simulink model "CTC"  (R2022b)
settings: Solver=VariableStepAuto  StartTime=0.0  StopTime=30  RelTol=1e-3
model workspace (MATLAB code in the model file):
  | % Simscape(TM) Multibody(TM) version: 7.3
  | 
  | % This is a model data file derived from a Simscape Multibody Import XML file using the smimport function.
  | % The data in this file sets the block parameter values in an imported Simscape Multibody model.
  | % For more information on this file, see the smimport function help page in the Simscape Multibody documentation.
  | % You can modify numerical values, but avoid any other changes to this file.
  | % Do not add code to this file. Do not edit the physical units shown in comments.
  | 
  | %%%VariableName:smiData
  | 
  | 
  | %============= RigidTransform =============%
  | 
  | %Initialize the RigidTransform structure array by filling in null values.
  | smiData.RigidTransform(98).translation = [0.0 0.0 0.0];
  | smiData.RigidTransform(98).angle = 0.0;
  | smiData.RigidTransform(98).axis = [0.0 0.0 0.0];
  | smiData.RigidTransform(98).ID = '';
  | 
  | %Translation Method - Cartesian
  | %Rotation Method - Arbitrary Axis
  | smiData.RigidTransform(1).translation = [0 19.999999999999989 175];  % mm
  | smiData.RigidTransform(1).angle = 2.0943951023931953;  % rad
  | smiData.RigidTransform(1).axis = [0.57735026918962584 -0.57735026918962584 0.57735026918962584];
  | smiData.RigidTransform(1).ID = 'B[UpperLeg_2:Upper_Leg-1:-:UpperLeg_2:Joint_1-1]';
  | 
  | %Translation Method - Cartesian
  | %Rotation Method - Arbitrary Axis
  | smiData.RigidTransform(2).translation = [-10.000000000089699 -1.8161827597396041e-10 -1.8518164779379731e-10];  % mm
  | smiData.RigidTransform(2).angle = 2.0943951023931953;  % rad
  | smiData.RigidTransform(2).axis = [0.57735026918962618 0.57735026918962562 0.5773502691896254];
  | smiData.RigidTransform(2).ID = 'F[UpperLeg_2:Upper_Leg-1:-:UpperLeg_2:Joint_1-1]';
  | 
  | %Translation Method - Cartesian
  | %Rotation Method - Arbitrary Axis
  | smiData.RigidTransform(3).translation = [117.00317547305409 9.9999999999999947 -56.489637028919212];  % mm
  | smiData.RigidTransform(3).angle = 0.52359877559830381;  % rad
  | smiData.RigidTransform(3).axis = [-0 -1 0];
  | smiData.RigidTransform(3).ID = 'B[Base_3:�?-1:-:Base_3:Joint_1-1]';
  | 
  | %Translation Method - Cartesian
  | %Rotation Method - Arbitrary Axis
  | smiData.RigidTransform(4).translation = [107.42304845737816 8.9706091443986224e-09 1.015528994230408e-08];  % mm
  | smiData.RigidTransform(4).angle = 2.0943951023930776;  % rad
  | smiData.RigidTransform(4).axis = [-0.57735026918962873 -0.57735026918958643 0.57735026918966204];
  | smiData.RigidTransform(4).ID = 'F[Base_3:�?-1:-:Base_3:Joint_1-1]';
  | 
  | %Translation Method - Cartesian
  | %Rotation Method - Arbitrary Axis
  | smiData.RigidTransform(5).translation = [-21.650635094607303 9.9999999999995097 108.66580753731172];  % mm
  | smiData.RigidTransform(5).angle = 3.1415926535897865;  % rad
  | smiData.RigidTransform(5).axis = [-0.96592582628906776 -8.8781377035549872e-16 0.25881904510252285];
  | smiData.RigidTransform(5).ID = 'B[Base_3:�?-1:-:Base_3:Joint_1-4]';
  | 
  | %Translation Method - Cartesian
  | %Rotation Method - Arbitrary Axis
  | smiData.RigidTransform(6).translation = [83.282032288587871 4.5821799687928433e-09 1.1489191820146516e-09];  % mm
  | smiData.RigidTransform(6).angle = 2.094395102393289;  % rad
  | smiData.RigidTransform(6).axis = [-0.57735026918951493 -0.57735026918965693 0.57735026918970545];
  | smiData.RigidTransform(6).ID = 'F[Base_3:�?-1:-:Base_3:Joint_1-4]';
  | 
  | %Translation Method - Cartesian
  | %Rotation Method - Arbitrary Axis
  | smiData.RigidTransform(7).translation = [-76.282032302753606 10.000000000000147 -73.082903768653054];  % mm
  | smiData.RigidTransform(7).angle = 2.094395102393197;  % rad
  | smiData.RigidTransform(7).axis = [0.57735026918962462 0.57735026918962629 0.5773502691896264];
  | smiData.RigidTransform(7).ID = 'B[Base_3:�?-1:-:Base_3:Joint_1-5]';
  | 
  | %Translation Method - Cartesian
  | %Rotation Method - Arbitrary Axis
  | smiData.RigidTransform(8).translation = [-76.28203231342502 8.5679736105508616e-09 -5.5658047997319685e-09];  % mm
  | smiData.RigidTransform(8).angle = 2.0943951023931096;  % rad
  | smiData.RigidTransform(8).axis = [0.57735026918957733 0.5773502691895972 0.57735026918970267];
  | smiData.RigidTransform(8).ID = 'F[Base_3:�?-1:-:Base_3:Joint_1-5]';
  | 
  | %Translation Method - Cartesian
  | %Rotation Method - Arbitrary Axis
  | smiData.RigidTransform(9).translation = [-18.655092795423545 178.99125127896585 252.03989417796402];  % mm
  | smiData.RigidTransform(9).angle = 2.094395102393197;  % rad
  | smiData.RigidTransform(9).axis = [0.5773502691896264 -0.57735026918962462 0.5773502691896264];
  | smiData.RigidTransform(9).ID = 'B[LowerLeg_Assembly#2-2:-:x?-10]';
  | 
  | %Translation Method - Cartesian
  | %Rotation Method - Arbitrary Axis
  | smiData.RigidTransform(10).translation = [3.0000000000001261 -4.0059067174524898e-12 -5.8264504332328215e-13];  % mm
  | smiData.RigidTransform(10).angle = 2.0943951023931953;  % rad
  | smiData.RigidTransform(10).axis = [0.57735026918962584 0.57735026918962584 0.57735026918962584];
  | smiData.RigidTransform(10).ID = 'F[LowerLeg_Assembly#2-2:-:x?-10]';
  | 
  | %Translation Method - Cartesian
  | %Rotation Method - Arbitrary Axis
  | smiData.RigidTransform(11).translation = [0 5.0000000000000044 0];  % mm
  | smiData.RigidTransform(11).angle = 2.0943951023931957;  % rad
  | smiData.RigidTransform(11).axis = [-0.57735026918962584 -0.57735026918962573 -0.57735026918962573];
  | smiData.RigidTransform(11).ID = 'B[UpperLeg_2-3:Joint_1-1:-:x?-10]';
  | 
  | %Translation Method - Cartesian
  | %Rotation Method - Arbitrary Axis
  | smiData.RigidTransform(12).translation = [-1.2569500995596172e-11 5.2091847198853705 -31.573159401015047];  % mm
  | smiData.RigidTransform(12).angle = 2.0943951023870682;  % rad
  | smiData.RigidTransform(12).axis = [-0.5773502691928436 -0.57735026918758314 0.57735026918845045];
  | smiData.RigidTransform(12).ID = 'F[UpperLeg_2-3:Joint_1-1:-:x?-10]';
  | 
  | %Translation Method - Cartesian
  | %Rotation Method - Arbitrary Axis
  | smiData.RigidTransform(13).translation = [31.999999999999918 5.0000000000000044 0];  % mm
  | smiData.RigidTransform(13).angle = 2.0943951023931953;  % rad
  | smiData.RigidTransform(13).axis = [0.57735026918962584 -0.57735026918962584 0.57735026918962584];
  | smiData.RigidTransform(13).ID = 'B[UpperLeg_2-5:Joint_1-1:-:x?-11]';
  | 
  | %Translation Method - Cartesian
  | %Rotation Method - Arbitrary Axis
  | smiData.RigidTransform(14).translation = [-7.9273054803145348e-11 1.3585044680166562e-11 -8.760761212378511e-11];  % mm
  | smiData.RigidTransform(14).angle = 2.0943951023967697;  % rad
  | smiData.RigidTransform(14).axis = [0.5773502691867648 0.57735026919081722 0.57735026919129528];
  | smiData.RigidTransform(14).ID = 'F[UpperLeg_2-5:Joint_1-1:-:x?-11]';
  | 
  | %Translation Method - Cartesian
  | %Rotation Method - Arbitrary Axis
  | smiData.RigidTransform(15).translation = [-32.000000000000028 5.0000000000000044 0];  % mm
  | smiData.RigidTransform(15).angle = 2.0943951023931953;  % rad
  | smiData.RigidTransform(15).axis = [0.57735026918962584 -0.57735026918962584 0.57735026918962584];
  | smiData.RigidTransform(15).ID = 'B[UpperLeg_2-5:Joint_1-1:-:x?-12]';
  | 
  | %Translation Method - Cartesian
  | %Rotation Method - Arbitrary Axis
  | smiData.RigidTransform(16).translation = [-7.9191762745372911e-11 1.3376425944582028e-11 -8.7773195960719397e-11];  % mm
  | smiData.RigidTransform(16).angle = 2.0943951023967693;  % rad
  | smiData.RigidTransform(16).axis = [0.57735026918676491 0.57735026919081711 0.57735026919129517];
  | smiData.RigidTransform(16).ID = 'F[UpperLeg_2-5:Joint_1-1:-:x?-12]';
  | 
  | %Translation Method - Cartesian
  | %Rotation Method - Arbitrary Axis
  | smiData.RigidTransform(17).translation = [130.75000000000338 55.000000000000355 -100.89195954089351];  % mm
  | smiData.RigidTransform(17).angle = 3.1415926535897878;  % rad
  | smiData.RigidTransform(17).axis = [0.96592582628906765 -7.5033484398435492e-16 -0.25881904510252302];
  | smiData.RigidTransform(17).ID = 'B[Base-1:-:UpperLeg_2-5:Upper_Leg-1]';
  | 
  | %Translation Method - Cartesian
  | %Rotation Method - Arbitrary Axis
  | smiData.RigidTransform(18).translation = [6.2172489379008766e-15 -12.000000000004182 -6.5725203057809267e-14];  % mm
  | smiData.RigidTransform(18).angle = 2.094395102393197;  % rad
  | smiData.RigidTransform(18).axis = [0.57735026918962629 -0.5773502691896254 0.57735026918962562];
  | smiData.RigidTransform(18).ID = 'F[Base-1:-:UpperLeg_2-5:Upper_Leg-1]';
  | 
  | %Translation Method - Cartesian
  | %Rotation Method - Arbitrary Axis
  | smiData.RigidTransform(19).translation = [353.38874943283707 174.99125127896704 252.03989417796384];  % mm
  | smiData.RigidTransform(19).angle = 2.0943951023931939;  % rad
  | smiData.RigidTransform(19).axis = [-0.57735026918962529 -0.57735026918962695 -0.57735026918962518];
  | smiData.RigidTransform(19).ID = 'B[LowerLeg_Assembly#2-1:-:Base_3-1:Joint_1-5]';
  | 
  | %Translation Method - Cartesian
  | %Rotation Method - Arbitrary Axis
  | smiData.RigidTransform(20).translation = [-32.00000001037607 2.0000000085989118 -5.446665340969048e-09];  % mm
  | smiData.RigidTransform(20).angle = 2.09439510239261;  % rad
  | smiData.RigidTransform(20).axis = [0.57735026918943078 -0.57735026918942933 0.5773502691900172];
  | smiData.RigidTransform(20).ID = 'F[LowerLeg_Assembly#2-1:-:Base_3-1:Joint_1-5]';
  | 
  | %Translation Method - Cartesian
  | %Rotation Method - Arbitrary Axis
  | smiData.RigidTransform(21).translation = [-32.000000000000028 5.000000000000032 0];  % mm
  | smiData.RigidTransform(21).angle = 2.0943951023931953;  % rad
  | smiData.RigidTransform(21).axis = [0.57735026918962584 -0.57735026918962584 0.57735026918962584];
  | smiData.RigidTransform(21).ID = 'B[UpperLeg_2-3:Joint_1-1:-:LowerLeg_Assembly#2-1]';
  | 
  | %Translation Method - Cartesian
  | %Rotation Method - Arbitrary Axis
  | smiData.RigidTransform(22).translation = [-18.655092795320627 181.99125127897832 252.03989417784715];  % mm
  | smiData.RigidTransform(22).angle = 2.0943951023881247;  % rad
  | smiData.RigidTransform(22).axis = [0.57735026918793542 -0.57735026919325916 0.57735026918768262];
  | smiData.RigidTransform(22).ID = 'F[UpperLeg_2-3:Joint_1-1:-:LowerLeg_Assembly#2-1]';
  | 
  | %Translation Method - Cartesian
  | %Rotation Method - Arbitrary Axis
  | smiData.RigidTransform(23).translation = [353.38874943283662 174.99125127896701 252.03989417796402];  % mm
  | smiData.RigidTransform(23).angle = 2.0943951023931939;  % rad
  | smiData.RigidTransform(23).axis = [-0.57735026918962529 -0.57735026918962706 -0.57735026918962495];
  | smiData.RigidTransform(23).ID = 'B[LowerLeg_Assembly#2-2:-:Base_3-1:Joint_1-5]';
  | 
  | %Translation Method - Cartesian
  | %Rotation Method - Arbitrary Axis
  | smiData.RigidTransform(24).translation = [31.999999989623838 2.000000008599276 -5.4573305874328071e-09];  % mm
  | smiData.RigidTransform(24).angle = 2.0943951023926095;  % rad
  | smiData.RigidTransform(24).axis = [0.57735026918943044 -0.57735026918942922 0.57735026919001764];
  | smiData.RigidTransform(24).ID = 'F[LowerLeg_Assembly#2-2:-:Base_3-1:Joint_1-5]';
  | 
  | %Translation Method - Cartesian
  | %Rotation Method - Arbitrary Axis
  | smiData.RigidTransform(25).translation = [31.999999999999972 5.000000000000032 0];  % mm
  | smiData.RigidTransform(25).angle = 2.0943951023931953;  % rad
  | smiData.RigidTransform(25).axis = [0.57735026918962584 -0.57735026918962584 0.57735026918962584];
  | smiData.RigidTransform(25).ID = 'B[UpperLeg_2-3:Joint_1-1:-:LowerLeg_Assembly#2-2]';
  | 
  | %Translation Method - Cartesian
  | %Rotation Method - Arbitrary Axis
  | smiData.RigidTransform(26).translation = [-18.655092795316818 181.99125127897861 252.03989417784709];  % mm
  | smiData.RigidTransform(26).angle = 2.0943951023881242;  % rad
  | smiData.RigidTransform(26).axis = [0.57735026918793531 -0.57735026919325916 0.57735026918768284];
  | smiData.RigidTransform(26).ID = 'F[UpperLeg_2-3:Joint_1-1:-:LowerLeg_Assembly#2-2]';
  | 
  | %Translation Method - Cartesian
  | %Rotation Method - Arbitrary Axis
  | smiData.RigidTransform(27).translation = [-18.655092795423545 174.99125127896542 252.03989417796402];  % mm
  | smiData.RigidTransform(27).angle = 2.0943951023931935;  % rad
  | smiData.RigidTransform(27).axis = [-0.57735026918962518 -0.57735026918962695 -0.57735026918962518];
  | smiData.RigidTransform(27).ID = 'B[LowerLeg_Assembly#2-3:-:Base_3-1:Joint_1-4]';
  | 
  | %Translation Method - Cartesian
  | %Rotation Method - Arbitrary Axis
  | smiData.RigidTransform(28).translation = [31.999999986078205 -1.9999999955871002 8.734324374870539e-10];  % mm
  | smiData.RigidTransform(28).angle = 2.094395102390521;  % rad
  | smiData.RigidTransform(28).axis = [-0.57735026918873433 -0.57735026918873378 -0.5773502691914093];
  | smiData.RigidTransform(28).ID = 'F[LowerLeg_Assembly#2-3:-:Base_3-1:Joint_1-4]';
  | 
  | %Translation Method - Cartesian
  | %Rotation Method - Arbitrary Axis
  | smiData.RigidTransform(29).translation = [-31.999999999999972 4.9999999999998934 0];  % mm
  | smiData.RigidTransform(29).angle = 2.0943951023931953;  % rad
  | smiData.RigidTransform(29).axis = [0.57735026918962584 -0.57735026918962584 0.57735026918962584];
  | smiData.RigidTransform(29).ID = 'B[UpperLeg_2-4:Joint_1-1:-:LowerLeg_Assembly#2-3]';
  | 
  | %Translation Method - Cartesian
  | %Rotation Method - Arbitrary Axis
  | smiData.RigidTransform(30).translation = [353.38874943270537 181.99125127899549 252.03989417800804];  % mm
  | smiData.RigidTransform(30).angle = 2.0943951023971508;  % rad
  | smiData.RigidTransform(30).axis = [0.57735026919094412 -0.57735026918594667 0.5773502691919864];
  | smiData.RigidTransform(30).ID = 'F[UpperLeg_2-4:Joint_1-1:-:LowerLeg_Assembly#2-3]';
  | 
  | %Translation Method - Cartesian
  | %Rotation Method - Arbitrary Axis
  | smiData.RigidTransform(31).translation = [-18.655092795423602 174.99125127896565 252.03989417796413];  % mm
  | smiData.RigidTransform(31).angle = 2.0943951023931935;  % rad
  | smiData.RigidTransform(31).axis = [-0.57735026918962518 -0.57735026918962695 -0.57735026918962518];
  | smiData.RigidTransform(31).ID = 'B[LowerLeg_Assembly#2-4:-:Base_3-1:Joint_1-4]';
  | 
  | %Translation Method - Cartesian
  | %Rotation Method - Arbitrary Axis
  | smiData.RigidTransform(32).translation = [-32.000000013922282 -1.9999999955870065 8.6944784705167422e-10];  % mm
  | smiData.RigidTransform(32).angle = 2.094395102390521;  % rad
  | smiData.RigidTransform(32).axis = [-0.57735026918873411 -0.57735026918873411 -0.57735026919140886];
  | smiData.RigidTransform(32).ID = 'F[LowerLeg_Assembly#2-4:-:Base_3-1:Joint_1-4]';
  | 
  | %Translation Method - Cartesian
  | %Rotation Method - Arbitrary Axis
  | smiData.RigidTransform(33).translation = [32.000000000000028 -4.5000000000001705 0];  % mm
  | smiData.RigidTransform(33).angle = 2.0943951023931953;  % rad
  | smiData.RigidTransform(33).axis = [0.57735026918962584 -0.57735026918962584 0.57735026918962584];
  | smiData.RigidTransform(33).ID = 'B[UpperLeg_2-4:Joint_1-1:-:LowerLeg_Assembly#2-4]';
  | 
  | %Translation Method - Cartesian
  | %Rotation Method - Arbitrary Axis
  | smiData.RigidTransform(34).translation = [353.38874943278768 172.49125127899504 252.03989417802512];  % mm
  | smiData.RigidTransform(34).angle = 2.0943951023971494;  % rad
  | smiData.RigidTransform(34).axis = [0.57735026919094379 -0.57735026918594712 0.57735026919198651];
  | smiData.RigidTransform(34).ID = 'F[UpperLeg_2-4:Joint_1-1:-:LowerLeg_Assembly#2-4]';
  | 
  | %Translation Method - Cartesian
  | %Rotation Method - Arbitrary Axis
  | smiData.RigidTransform(35).translation = [-18.655092795423659 174.99125127896588 252.03989417796402];  % mm
  | smiData.RigidTransform(35).angle = 2.0943951023931935;  % rad
  | smiData.RigidTransform(35).axis = [-0.57735026918962518 -0.57735026918962695 -0.57735026918962518];
  | smiData.RigidTransform(35).ID = 'B[LowerLeg_Assembly#2-5:-:Base_3-1:Joint_1-1]';
  | 
  | %Translation Method - Cartesian
  | %Rotation Method - Arbitrary Axis
  | smiData.RigidTransform(36).translation = [-31.999999996925382 2.0000000089001038 9.9767270000938879e-09];  % mm
  | smiData.RigidTransform(36).angle = 2.0943951023932001;  % rad
  | smiData.RigidTransform(36).axis = [0.57735026918962729 -0.57735026918962384 0.57735026918962629];
  | smiData.RigidTransform(36).ID = 'F[LowerLeg_Assembly#2-5:-:Base_3-1:Joint_1-1]';
  | 
  | %Translation Method - Cartesian
  | %Rotation Method - Arbitrary Axis
  | smiData.RigidTransform(37).translation = [-18.655092795423542 174.99125127896585 252.03989417796407];  % mm
  | smiData.RigidTransform(37).angle = 2.0943951023931935;  % rad
  | smiData.RigidTransform(37).axis = [-0.57735026918962518 -0.57735026918962695 -0.57735026918962518];
  | smiData.RigidTransform(37).ID = 'B[LowerLeg_Assembly#2-6:-:Base_3-1:Joint_1-1]';
  | 
  | %Translation Method - Cartesian
  | %Rotation Method - Arbitrary Axis
  | smiData.RigidTransform(38).translation = [32.000000003094932 2.0000000089002699 1.0007141781898099e-08];  % mm
  | smiData.RigidTransform(38).angle = 2.0943951023932006;  % rad
  | smiData.RigidTransform(38).axis = [0.5773502691896274 -0.5773502691896244 0.57735026918962551];
  | smiData.RigidTransform(38).ID = 'F[LowerLeg_Assembly#2-6:-:Base_3-1:Joint_1-1]';
  | 
  | %Translation Method - Cartesian
  | %Rotation Method - Arbitrary Axis
  | smiData.RigidTransform(39).translation = [-7.9999999999974776 54.999999999999467 163.67880131526533];  % mm
  | smiData.RigidTransform(39).angle = 2.0943951023931975;  % rad
  | smiData.RigidTransform(39).axis = [-0.57735026918962351 -0.57735026918962651 0.57735026918962717];
  | smiData.RigidTransform(39).ID = 'B[Base-1:-:UpperLeg_2-4:Upper_Leg-1]';
  | 
  | %Translation Method - Cartesian
  | %Rotation Method - Arbitrary Axis
  | smiData.RigidTransform(40).translation = [-2.6645352591003757e-15 2 -1.6620038678638593e-13];  % mm
  | smiData.RigidTransform(40).angle = 2.0943951023931953;  % rad
  | smiData.RigidTransform(40).axis = [0.57735026918962584 -0.57735026918962595 0.57735026918962562];
  | smiData.RigidTransform(40).ID = 'F[Base-1:-:UpperLeg_2-4:Upper_Leg-1]';
  | 
  | %Translation Method - Cartesian
  | %Rotation Method - Arbitrary Axis
  | smiData.RigidTransform(41).translation = [-137.75000000000676 54.999999999998977 -88.767603887906532];  % mm
  | smiData.RigidTransform(41).angle = 3.1415926535897931;  % rad
  | smiData.RigidTransform(41).axis = [-0.96592582628906787 2.1099173714894905e-17 -0.25881904510252235];
  | smiData.RigidTransform(41).ID = 'B[Base-1:-:UpperLeg_2-3:Upper_Leg-1]';
  | 
  | %Translation Method - Cartesian
  | %Rotation Method - Arbitrary Axis
  | smiData.RigidTransform(42).translation = [5.4622972811557702e-14 1.9999999999999671 -1.6431300764452317e-14];  % mm
  | smiData.RigidTransform(42).angle = 2.0943951023931953;  % rad
  | smiData.RigidTransform(42).axis = [0.57735026918962584 -0.57735026918962551 0.57735026918962606];
  | smiData.RigidTransform(42).ID = 'F[Base-1:-:UpperLeg_2-3:Upper_Leg-1]';
  | 
  | %Translation Method - Cartesian
  | %Rotation Method - Arbitrary Axis
  | smiData.RigidTransform(43).translation = [-32.000000000000028 5.0000000000000044 0];  % mm
  | smiData.RigidTransform(43).angle = 2.0943951023931953;  % rad
  | smiData.RigidTransform(43).axis = [0.57735026918962584 -0.57735026918962584 0.57735026918962584];
  | smiData.RigidTransform(43).ID = 'B[UpperLeg_2-5:Joint_1-1:-:LowerLeg_Assembly#2-5]';
  | 
  | %Translation Method - Cartesian
  | %Rotation Method - Arbitrary Axis
  | smiData.RigidTransform(44).translation = [353.3887494325952 171.99125127888766 252.0398941777938];  % mm
  | smiData.RigidTransform(44).angle = 2.0943951023885226;  % rad
  | smiData.RigidTransform(44).axis = [-0.57735026918806809 -0.57735026919209964 -0.57735026918870969];
  | smiData.RigidTransform(44).ID = 'F[UpperLeg_2-5:Joint_1-1:-:LowerLeg_Assembly#2-5]';
  | 
  | %Translation Method - Cartesian
  | %Rotation Method - Arbitrary Axis
  | smiData.RigidTransform(45).translation = [31.999999999999918 5.0000000000000044 0];  % mm
  | smiData.RigidTransform(45).angle = 2.0943951023931953;  % rad
  | smiData.RigidTransform(45).axis = [0.57735026918962584 -0.57735026918962584 0.57735026918962584];
  | smiData.RigidTransform(45).ID = 'B[UpperLeg_2-5:Joint_1-1:-:LowerLeg_Assembly#2-6]';
  | 
  | %Translation Method - Cartesian
  | %Rotation Method - Arbitrary Axis
  | smiData.RigidTransform(46).translation = [353.38874943263181 171.99125127888817 252.03989417779786];  % mm
  | smiData.RigidTransform(46).angle = 2.0943951023885221;  % rad
  | smiData.RigidTransform(46).axis = [-0.57735026918806798 -0.57735026919210009 -0.57735026918870913];
  | smiData.RigidTransform(46).ID = 'F[UpperLeg_2-5:Joint_1-1:-:LowerLeg_Assembly#2-6]';
  | 
  | %Translation Method - Cartesian
  | %Rotation Method - Arbitrary Axis
  | smiData.RigidTransform(47).translation = [-31.999999999999972 4.9999999999998934 0];  % mm
  | smiData.RigidTransform(47).angle = 2.0943951023931953;  % rad
  | smiData.RigidTransform(47).axis = [0.57735026918962584 -0.57735026918962584 0.57735026918962584];
  | smiData.RigidTransform(47).ID = 'B[UpperLeg_2-4:Joint_1-1:-:x?-1]';
  | 
  | %Translation Method - Cartesian
  | %Rotation Method - Arbitrary Axis
  | smiData.RigidTransform(48).translation = [-2.8304693339204936e-11 8.1275372056386725e-11 -1.1228050902199318e-10];  % mm
  | smiData.RigidTransform(48).angle = 2.0943951023864673;  % rad
  | smiData.RigidTransform(48).axis = [0.57735026919205323 0.57735026918738308 0.5773502691894411];
  | smiData.RigidTransform(48).ID = 'F[UpperLeg_2-4:Joint_1-1:-:x?-1]';
  | 
  | %Translation Method - Cartesian
  | %Rotation Method - Arbitrary Axis
  | smiData.RigidTransform(49).translation = [353.3887494328369 174.99125127896721 252.03989417796407];  % mm
  | smiData.RigidTransform(49).angle = 2.0943951023931939;  % rad
  | smiData.RigidTransform(49).axis = [-0.57735026918962529 -0.57735026918962695 -0.57735026918962518];
  | smiData.RigidTransform(49).ID = 'B[LowerLeg_Assembly#2-4:-:x?-2]';
  | 
  | %Translation Method - Cartesian
  | %Rotation Method - Arbitrary Axis
  | smiData.RigidTransform(50).translation = [3.0000000000004716 1.5765166949677223e-14 3.0020430585864233e-13];  % mm
  | smiData.RigidTransform(50).angle = 2.094395102393197;  % rad
  | smiData.RigidTransform(50).axis = [0.57735026918962506 0.57735026918962629 0.57735026918962606];
  | smiData.RigidTransform(50).ID = 'F[LowerLeg_Assembly#2-4:-:x?-2]';
  | 
  | %Translation Method - Cartesian
  | %Rotation Method - Arbitrary Axis
  | smiData.RigidTransform(51).translation = [0 4.9999999999998934 0];  % mm
  | smiData.RigidTransform(51).angle = 2.0943951023931953;  % rad
  | smiData.RigidTransform(51).axis = [-0.57735026918962584 -0.57735026918962584 -0.57735026918962584];
  | smiData.RigidTransform(51).ID = 'B[UpperLeg_2-4:Joint_1-1:-:x?-2]';
  | 
  | %Translation Method - Cartesian
  | %Rotation Method - Arbitrary Axis
  | smiData.RigidTransform(52).translation = [10.000000000028464 -18.871620680049485 -25.843024840444919];  % mm
  | smiData.RigidTransform(52).angle = 2.0943951024003273;  % rad
  | smiData.RigidTransform(52).axis = [0.57735026918788079 0.57735026919200305 0.57735026918899346];
  | smiData.RigidTransform(52).ID = 'F[UpperLeg_2-4:Joint_1-1:-:x?-2]';
  | 
  | %Translation Method - Cartesian
  | %Rotation Method - Arbitrary Axis
  | smiData.RigidTransform(53).translation = [-18.655092795423602 174.99125127896565 252.03989417796413];  % mm
  | smiData.RigidTransform(53).angle = 2.0943951023931935;  % rad
  | smiData.RigidTransform(53).axis = [-0.57735026918962518 -0.57735026918962695 -0.57735026918962518];
  | smiData.RigidTransform(53).ID = 'B[LowerLeg_Assembly#2-4:-:x?-3]';
  | 
  | %Translation Method - Cartesian
  | %Rotation Method - Arbitrary Axis
  | smiData.RigidTransform(54).translation = [2.9999999999996385 1.2345680033831741e-13 5.9063864910058328e-14];  % mm
  | smiData.RigidTransform(54).angle = 2.0943951023931957;  % rad
  | smiData.RigidTransform(54).axis = [0.57735026918962573 0.57735026918962584 0.57735026918962573];
  | smiData.RigidTransform(54).ID = 'F[LowerLeg_Assembly#2-4:-:x?-3]';
  | 
  | %Translation Method - Cartesian
  | %Rotation Method - Arbitrary Axis
  | smiData.RigidTransform(55).translation = [0 4.9999999999998934 0];  % mm
  | smiData.RigidTransform(55).angle = 2.0943951023931953;  % rad
  | smiData.RigidTransform(55).axis = [-0.57735026918962584 -0.57735026918962584 -0.57735026918962584];
  | smiData.RigidTransform(55).ID = 'B[Base_3-1:Joint_1-4:-:x?-3]';
  | 
  | %Translation Method - Cartesian
  | %Rotation Method - Arbitrary Axis
  | smiData.RigidTransform(56).translation = [9.9999999955865597 -18.871620687174598 -25.84302485256751];  % mm
  | smiData.RigidTransform(56).angle = 2.094395102396934;  % rad
  | smiData.RigidTransform(56).axis = [0.57735026918871135 0.57735026919087207 0.57735026918929389];
  | smiData.RigidTransform(56).ID = 'F[Base_3-1:Joint_1-4:-:x?-3]';
  | 
  | %Translation Method - Cartesian
  | %Rotation Method - Arbitrary Axis
  | smiData.RigidTransform(57).translation = [32 2.0000000000000018 0];  % mm
  | smiData.RigidTransform(57).angle = 2.0943951023931953;  % rad
  | smiData.RigidTransform(57).axis = [-0.57735026918962584 -0.57735026918962584 -0.57735026918962584];
  | smiData.RigidTransform(57).ID = 'B[Base_3-1:Joint_1-4:-:x?-4]';
  | 
  | %Translation Method - Cartesian
  | %Rotation Method - Arbitrary Axis
  | smiData.RigidTransform(58).translation = [6.9999999955868182 -4.7997881225114725e-09 -1.3098889084517396e-08];  % mm
  | smiData.RigidTransform(58).angle = 2.0943951023967227;  % rad
  | smiData.RigidTransform(58).axis = [0.57735026918835308 0.57735026919080146 0.57735026918972265];
  | smiData.RigidTransform(58).ID = 'F[Base_3-1:Joint_1-4:-:x?-4]';
  | 
  | %Translation Method - Cartesian
  | %Rotation Method - Arbitrary Axis
  | smiData.RigidTransform(59).translation = [-32.000000000000028 5.0000000000000044 0];  % mm
  | smiData.RigidTransform(59).angle = 2.0943951023931953;  % rad
  | smiData.RigidTransform(59).axis = [0.57735026918962584 -0.57735026918962584 0.57735026918962584];
  | smiData.RigidTransform(59).ID = 'B[Base_3-1:Joint_1-1:-:x?-5]';
  | 
  | %Translation Method - Cartesian
  | %Rotation Method - Arbitrary Axis
  | smiData.RigidTransform(60).translation = [8.8995385915898682e-09 -1.0387659761905275e-08 1.9259925562826736e-09];  % mm
  | smiData.RigidTransform(60).angle = 2.094395102393193;  % rad
  | smiData.RigidTransform(60).axis = [0.57735026918962429 0.57735026918962506 0.57735026918962806];
  | smiData.RigidTransform(60).ID = 'F[Base_3-1:Joint_1-1:-:x?-5]';
  | 
  | %Translation Method - Cartesian
  | %Rotation Method - Arbitrary Axis
  | smiData.RigidTransform(61).translation = [32.000000000000028 4.9999999999998934 -1.1102230246251565e-13];  % mm
  | smiData.RigidTransform(61).angle = 2.0943951023931953;  % rad
  | smiData.RigidTransform(61).axis = [0.57735026918962584 -0.57735026918962584 0.57735026918962584];
  | smiData.RigidTransform(61).ID = 'B[Base_3-1:Joint_1-1:-:x?-6]';
  | 
  | %Translation Method - Cartesian
  | %Rotation Method - Arbitrary Axis
  | smiData.RigidTransform(62).translation = [8.9002074097319125e-09 -1.0387637321704619e-08 1.9258838674308523e-09];  % mm
  | smiData.RigidTransform(62).angle = 2.0943951023931935;  % rad
  | smiData.RigidTransform(62).axis = [0.57735026918962418 0.57735026918962506 0.57735026918962806];
  | smiData.RigidTransform(62).ID = 'F[Base_3-1:Joint_1-1:-:x?-6]';
  | 
  | %Translation Method - Cartesian
  | %Rotation Method - Arbitrary Axis
  | smiData.RigidTransform(63).translation = [-31.999999999999972 4.9999999999999769 0];  % mm
  | smiData.RigidTransform(63).angle = 2.0943951023931953;  % rad
  | smiData.RigidTransform(63).axis = [0.57735026918962584 -0.57735026918962584 0.57735026918962584];
  | smiData.RigidTransform(63).ID = 'B[Base_3-1:Joint_1-5:-:x?-7]';
  | 
  | %Translation Method - Cartesian
  | %Rotation Method - Arbitrary Axis
  | smiData.RigidTransform(64).translation = [9.9999999923601948 -4.0414445123815312e-09 -1.1124877019597079e-08];  % mm
  | smiData.RigidTransform(64).angle = 2.0943951023931944;  % rad
  | smiData.RigidTransform(64).axis = [-0.57735026918962662 -0.57735026918962529 0.57735026918962529];
  | smiData.RigidTransform(64).ID = 'F[Base_3-1:Joint_1-5:-:x?-7]';
  | 
  | %Translation Method - Cartesian
  | %Rotation Method - Arbitrary Axis
  | smiData.RigidTransform(65).translation = [31.999999999999972 4.9999999999999769 0];  % mm
  | smiData.RigidTransform(65).angle = 2.0943951023931953;  % rad
  | smiData.RigidTransform(65).axis = [0.57735026918962584 -0.57735026918962584 0.57735026918962584];
  | smiData.RigidTransform(65).ID = 'B[Base_3-1:Joint_1-5:-:x?-8]';
  | 
  | %Translation Method - Cartesian
  | %Rotation Method - Arbitrary Axis
  | smiData.RigidTransform(66).translation = [9.9999999923605003 -4.041403656174225e-09 -1.1124982712829024e-08];  % mm
  | smiData.RigidTransform(66).angle = 2.0943951023931935;  % rad
  | smiData.RigidTransform(66).axis = [-0.5773502691896264 -0.57735026918962506 0.57735026918962584];
  | smiData.RigidTransform(66).ID = 'F[Base_3-1:Joint_1-5:-:x?-8]';
  | 
  | %Translation Method - Cartesian
  | %Rotation Method - Arbitrary Axis
  | smiData.RigidTransform(67).translation = [-32.000000000000028 5.000000000000032 0];  % mm
  | smiData.RigidTransform(67).angle = 2.0943951023931953;  % rad
  | smiData.RigidTransform(67).axis = [0.57735026918962584 -0.57735026918962584 0.57735026918962584];
  | smiData.RigidTransform(67).ID = 'B[UpperLeg_2-3:Joint_1-1:-:x?-9]';
  | 
  | %Translation Method - Cartesian
  | %Rotation Method - Arbitrary Axis
  | smiData.RigidTransform(68).translation = [5.7005566882496961e-10 -5.2147214954237031e-12 1.2153016596227291e-10];  % mm
  | smiData.RigidTransform(68).angle = 2.0943951023983431;  % rad
  | smiData.RigidTransform(68).axis = [0.57735026918546817 0.57735026919134169 0.57735026919206744];
  | smiData.RigidTransform(68).ID = 'F[UpperLeg_2-3:Joint_1-1:-:x?-9]';
  | 
  | %Translation Method - Cartesian
  | %Rotation Method - Arbitrary Axis
  | smiData.RigidTransform(69).translation = [317.36682831870667 176.99125127896687 252.03989417796384];  % mm
  | smiData.RigidTransform(69).angle = 3.1415926535897931;  % rad
  | smiData.RigidTransform(69).axis = [1 1.5785983631388952e-15 0];
  | smiData.RigidTransform(69).ID = 'AssemblyGround[LowerLeg_Assembly#2-1:Joint_2-2]';
  | 
  | %Translation Method - Cartesian
  | %Rotation Method - Arbitrary Axis
  | smiData.RigidTransform(70).translation = [167.36682831870652 176.99125127896701 252.0398941779639];  % mm
  | smiData.RigidTransform(70).angle = 0;  % rad
  | smiData.RigidTransform(70).axis = [0 0 0];
  | smiData.RigidTransform(70).ID = 'AssemblyGround[LowerLeg_Assembly#2-1:Lower_Leg-1]';
  | 
  | %Translation Method - Cartesian
  | %Rotation Method - Arbitrary Axis
  | smiData.RigidTransform(71).translation = [17.366828318706617 176.99125127896588 252.03989417796396];  % mm
  | smiData.RigidTransform(71).angle = 3.14159265358979;  % rad
  | smiData.RigidTransform(71).axis = [-0 5.5511151231257815e-17 -1];
  | smiData.RigidTransform(71).ID = 'AssemblyGround[LowerLeg_Assembly#2-1:Joint_2-1]';
  | 
  | %Translation Method - Cartesian
  | %Rotation Method - Arbitrary Axis
  | smiData.RigidTransform(72).translation = [317.36682831870655 176.99125127896696 252.03989417796402];  % mm
  | smiData.RigidTransform(72).angle = 3.1415926535897931;  % rad
  | smiData.RigidTransform(72).axis = [1 1.6306400674181995e-15 0];
  | smiData.RigidTransform(72).ID = 'AssemblyGround[LowerLeg_Assembly#2-2:Joint_2-2]';
  | 
  | %Translation Method - Cartesian
  | %Rotation Method - Arbitrary Axis
  | smiData.RigidTransform(73).translation = [167.36682831870652 176.99125127896696 252.03989417796396];  % mm
  | smiData.RigidTransform(73).angle = 0;  % rad
  | smiData.RigidTransform(73).axis = [0 0 0];
  | smiData.RigidTransform(73).ID = 'AssemblyGround[LowerLeg_Assembly#2-2:Lower_Leg-1]';
  | 
  | %Translation Method - Cartesian
  | %Rotation Method - Arbitrary Axis
  | smiData.RigidTransform(74).translation = [17.366828318706506 176.9912512789659 252.03989417796402];  % mm
  | smiData.RigidTransform(74).angle = 3.14159265358979;  % rad
  | smiData.RigidTransform(74).axis = [-0 -0 -1];
  | smiData.RigidTransform(74).ID = 'AssemblyGround[LowerLeg_Assembly#2-2:Joint_2-1]';
  | 
  | %Translation Method - Cartesian
  | %Rotation Method - Arbitrary Axis
  | smiData.RigidTransform(75).translation = [317.3668283187065 176.99125127896687 252.0398941779639];  % mm
  | smiData.RigidTransform(75).angle = 3.1415926535897931;  % rad
  | smiData.RigidTransform(75).axis = [1 1.5959455978986625e-15 0];
  | smiData.RigidTransform(75).ID = 'AssemblyGround[LowerLeg_Assembly#2-3:Joint_2-2]';
  | 
  | %Translation Method - Cartesian
  | %Rotation Method - Arbitrary Axis
  | smiData.RigidTransform(76).translation = [167.36682831870635 176.9912512789671 252.0398941779639];  % mm
  | smiData.RigidTransform(76).angle = 0;  % rad
  | smiData.RigidTransform(76).axis = [0 0 0];
  | smiData.RigidTransform(76).ID = 'AssemblyGround[LowerLeg_Assembly#2-3:Lower_Leg-1]';
  | 
  | %Translation Method - Cartesian
  | %Rotation Method - Arbitrary Axis
  | smiData.RigidTransform(77).translation = [17.36682831870645 176.99125127896576 252.03989417796402];  % mm
  | smiData.RigidTransform(77).angle = 3.1415926535897905;  % rad
  | smiData.RigidTransform(77).axis = [-0 -0 -1];
  | smiData.RigidTransform(77).ID = 'AssemblyGround[LowerLeg_Assembly#2-3:Joint_2-1]';
  | 
  | %Translation Method - Cartesian
  | %Rotation Method - Arbitrary Axis
  | smiData.RigidTransform(78).translation = [317.36682831870672 176.9912512789671 252.03989417796407];  % mm
  | smiData.RigidTransform(78).angle = 3.1415926535897931;  % rad
  | smiData.RigidTransform(78).axis = [1 1.5959455978986625e-15 0];
  | smiData.RigidTransform(78).ID = 'AssemblyGround[LowerLeg_Assembly#2-4:Joint_2-2]';
  | 
  | %Translation Method - Cartesian
  | %Rotation Method - Arbitrary Axis
  | smiData.RigidTransform(79).translation = [167.36682831870658 176.9912512789671 252.03989417796407];  % mm
  | smiData.RigidTransform(79).angle = 0;  % rad
  | smiData.RigidTransform(79).axis = [0 0 0];
  | smiData.RigidTransform(79).ID = 'AssemblyGround[LowerLeg_Assembly#2-4:Lower_Leg-1]';
  | 
  | %Translation Method - Cartesian
  | %Rotation Method - Arbitrary Axis
  | smiData.RigidTransform(80).translation = [17.366828318706506 176.99125127896599 252.03989417796413];  % mm
  | smiData.RigidTransform(80).angle = 3.14159265358979;  % rad
  | smiData.RigidTransform(80).axis = [-0 -0 -1];
  | smiData.RigidTransform(80).ID = 'AssemblyGround[LowerLeg_Assembly#2-4:Joint_2-1]';
  | 
  | %Translation Method - Cartesian
  | %Rotation Method - Arbitrary Axis
  | smiData.RigidTransform(81).translation = [-132.09936490539647 29.999999999999471 -48.554790966802265];  % mm
  | smiData.RigidTransform(81).angle = 2.0943951023931864;  % rad
  | smiData.RigidTransform(81).axis = [3.4416913763379853e-15 -1 -0];
  | smiData.RigidTransform(81).ID = 'AssemblyGround[Base-1:Gá_cho_Upper_Leg-6]';
  | 
  | %Translation Method - Cartesian
  | %Rotation Method - Arbitrary Axis
  | smiData.RigidTransform(82).translation = [-158.40063509461757 29.99999999999886 -102.99965469547534];  % mm
  | smiData.RigidTransform(82).angle = 1.0471975511965943;  % rad
  | smiData.RigidTransform(82).axis = [-5.1625370645069882e-15 1 2.9805921638945374e-15];
  | smiData.RigidTransform(82).ID = 'AssemblyGround[Base-1:Gá_cho_Upper_Leg-2]';
  | 
  | %Translation Method - Cartesian
  | %Rotation Method - Arbitrary Axis
  | smiData.RigidTransform(83).translation = [108.09936490539252 30.000000000000306 -90.124010348462178];  % mm
  | smiData.RigidTransform(83).angle = 2.0943951023932001;  % rad
  | smiData.RigidTransform(83).axis = [-3.4416913763379853e-15 1 2.6295363507366989e-31];
  | smiData.RigidTransform(83).ID = 'AssemblyGround[Base-1:Gá_cho_Upper_Leg-5]';
  | 
  | %Translation Method - Cartesian
  | %Rotation Method - Arbitrary Axis
  | smiData.RigidTransform(84).translation = [-9.9999999999972893 29.999999999999361 188.67880131526528];  % mm
  | smiData.RigidTransform(84).angle = 3.1415926535897918;  % rad
  | smiData.RigidTransform(84).axis = [2.5812685322534759e-15 -1 -1.4902960819472681e-15];
  | smiData.RigidTransform(84).ID = 'AssemblyGround[Base-1:Gá_cho_Upper_Leg-3]';
  | 
  | %Translation Method - Cartesian
  | %Rotation Method - Arbitrary Axis
  | smiData.RigidTransform(85).translation = [168.40063509461578 30.000000000000028 -85.679146619789151];  % mm
  | smiData.RigidTransform(85).angle = 1.0471975511966056;  % rad
  | smiData.RigidTransform(85).axis = [0 -1 0];
  | smiData.RigidTransform(85).ID = 'AssemblyGround[Base-1:Gá_cho_Upper_Leg-1]';
  | 
  | %Translation Method - Cartesian
  | %Rotation Method - Arbitrary Axis
  | smiData.RigidTransform(86).translation = [-349.99999999999716 0 202.07259421637502];  % mm
  | smiData.RigidTransform(86).angle = 0;  % rad
  | smiData.RigidTransform(86).axis = [0 0 0];
  | smiData.RigidTransform(86).ID = 'AssemblyGround[Base-1:M?t_Base-1]';
  | 
  | %Translation Method - Cartesian
  | %Rotation Method - Arbitrary Axis
  | smiData.RigidTransform(87).translation = [24.000000000002853 29.999999999999972 138.6788013152651];  % mm
  | smiData.RigidTransform(87).angle = 0;  % rad
  | smiData.RigidTransform(87).axis = [0 0 0];
  | smiData.RigidTransform(87).ID = 'AssemblyGround[Base-1:Gá_cho_Upper_Leg-4]';
  | 
  | %Translation Method - Cartesian
  | %Rotation Method - Arbitrary Axis
  | smiData.RigidTransform(88).translation = [317.36682831870661 176.99125127896698 252.0398941779639];  % mm
  | smiData.RigidTransform(88).angle = 3.1415926535897931;  % rad
  | smiData.RigidTransform(88).axis = [1 1.5820678100908481e-15 0];
  | smiData.RigidTransform(88).ID = 'AssemblyGround[LowerLeg_Assembly#2-5:Joint_2-2]';
  | 
  | %Translation Method - Cartesian
  | %Rotation Method - Arbitrary Axis
  | smiData.RigidTransform(89).translation = [167.36682831870641 176.9912512789671 252.0398941779639];  % mm
  | smiData.RigidTransform(89).angle = 0;  % rad
  | smiData.RigidTransform(89).axis = [0 0 0];
  | smiData.RigidTransform(89).ID = 'AssemblyGround[LowerLeg_Assembly#2-5:Lower_Leg-1]';
  | 
  | %Translation Method - Cartesian
  | %Rotation Method - Arbitrary Axis
  | smiData.RigidTransform(90).translation = [17.366828318706506 176.99125127896599 252.03989417796402];  % mm
  | smiData.RigidTransform(90).angle = 3.14159265358979;  % rad
  | smiData.RigidTransform(90).axis = [-0 2.7755575615628914e-17 -1];
  | smiData.RigidTransform(90).ID = 'AssemblyGround[LowerLeg_Assembly#2-5:Joint_2-1]';
  | 
  | %Translation Method - Cartesian
  | %Rotation Method - Arbitrary Axis
  | smiData.RigidTransform(91).translation = [317.36682831870655 176.9912512789671 252.03989417796407];  % mm
  | smiData.RigidTransform(91).angle = 3.1415926535897931;  % rad
  | smiData.RigidTransform(91).axis = [1 1.6202317265623378e-15 0];
  | smiData.RigidTransform(91).ID = 'AssemblyGround[LowerLeg_Assembly#2-6:Joint_2-2]';
  | 
  | %Translation Method - Cartesian
  | %Rotation Method - Arbitrary Axis
  | smiData.RigidTransform(92).translation = [167.36682831870641 176.99125127896721 252.03989417796396];  % mm
  | smiData.RigidTransform(92).angle = 0;  % rad
  | smiData.RigidTransform(92).axis = [0 0 0];
  | smiData.RigidTransform(92).ID = 'AssemblyGround[LowerLeg_Assembly#2-6:Lower_Leg-1]';
  | 
  | %Translation Method - Cartesian
  | %Rotation Method - Arbitrary Axis
  | smiData.RigidTransform(93).translation = [17.366828318706396 176.99125127896608 252.03989417796407];  % mm
  | smiData.RigidTransform(93).angle = 3.14159265358979;  % rad
  | smiData.RigidTransform(93).axis = [-0 -0 -1];
  | smiData.RigidTransform(93).ID = 'AssemblyGround[LowerLeg_Assembly#2-6:Joint_2-1]';
  | 
  | %Translation Method - Cartesian
  | %Rotation Method - Arbitrary Axis
  | smiData.RigidTransform(94).translation = [98.676365677353829 132.3022877755734 55.05600019288903];  % mm
  | smiData.RigidTransform(94).angle = 0;  % rad
  | smiData.RigidTransform(94).axis = [0 0 0];
  | smiData.RigidTransform(94).ID = 'AssemblyGround[UpperLeg_2-3:Upper_Leg-1]';
  | 
  | %Translation Method - Cartesian
  | %Rotation Method - Arbitrary Axis
  | smiData.RigidTransform(95).translation = [98.676365677353886 132.30228777557332 55.056000192889258];  % mm
  | smiData.RigidTransform(95).angle = 0;  % rad
  | smiData.RigidTransform(95).axis = [0 0 0];
  | smiData.RigidTransform(95).ID = 'AssemblyGround[UpperLeg_2-4:Upper_Leg-1]';
  | 
  | %Translation Method - Cartesian
  | %Rotation Method - Arbitrary Axis
  | smiData.RigidTransform(96).translation = [98.676365677353857 132.30228777557329 55.05600019288903];  % mm
  | smiData.RigidTransform(96).angle = 0;  % rad
  | smiData.RigidTransform(96).axis = [0 0 0];
  | smiData.RigidTransform(96).ID = 'AssemblyGround[UpperLeg_2-5:Upper_Leg-1]';
  | 
  | %Translation Method - Cartesian
  | %Rotation Method - Arbitrary Axis
  | smiData.RigidTransform(97).translation = [202.66916501977906 424.47951410922889 601.89799815844515];  % mm
  | smiData.RigidTransform(97).angle = 0;  % rad
  | smiData.RigidTransform(97).axis = [0 0 0];
  | smiData.RigidTransform(97).ID = 'RootGround[Base-1]';
  | 
  | %Translation Method - Cartesian
  | %Rotation Method - Arbitrary Axis
  | smiData.RigidTransform(98).translation = [73.455119007155062 73.362093584715467 123.44334172319465];  % mm
  | smiData.RigidTransform(98).angle = 0;  % rad
  | smiData.RigidTransform(98).axis = [0 0 0];
  | smiData.RigidTransform(98).ID = 'AssemblyGround[Base_3-1:�?-1]';
  | 
  | 
  | %============= Solid =============%
  | %Center of Mass (CoM) %Moments of Inertia (MoI) %Product of Inertia (PoI)
  | 
  | %Initialize the Solid structure array by filling in null values.
  | smiData.Solid(8).mass = 0.0;
  | smiData.Solid(8).CoM = [0.0 0.0 0.0];
  | smiData.Solid(8).MoI = [0.0 0.0 0.0];
  | smiData.Solid(8).PoI = [0.0 0.0 0.0];
  | smiData.Solid(8).color = [0.0 0.0 0.0];
  | smiData.Solid(8).opacity = 0.0;
  | smiData.Solid(8).ID = '';
  | 
  | %Inertia Type - Custom
  | %Visual Properties - Simple
  | smiData.Solid(1).mass = 0.14169795977416536;  % kg
  | smiData.Solid(1).CoM = [0 10 67.023520991164446];  % mm
  | smiData.Solid(1).MoI = [445.15612541920501 458.46395773552138 22.754362967927399];  % kg*mm^2
  | smiData.Solid(1).PoI = [0 0 0];  % kg*mm^2
  | smiData.Solid(1).color = [0.792156862745098 0.81960784313725488 0.93333333333333335];
  | smiData.Solid(1).opacity = 1;
  | smiData.Solid(1).ID = 'Upper_Leg*:*Default';
  | 
  | %Inertia Type - Custom
  | %Visual Properties - Simple
  | smiData.Solid(2).mass = 0.005037243917636585;  % kg
  | smiData.Solid(2).CoM = [-0.031113290901329776 0.0016751892373617883 0.004102426591954888];  % mm
  | smiData.Solid(2).MoI = [0.2179244214963923 4.5856280674254295 4.4704164196711993];  % kg*mm^2
  | smiData.Solid(2).PoI = [1.4371754332126697e-07 0.00066351909960837179 -0.00026944425684977087];  % kg*mm^2
  | smiData.Solid(2).color = [0.792156862745098 0.81960784313725488 0.93333333333333335];
  | smiData.Solid(2).opacity = 1;
  | smiData.Solid(2).ID = 'Joint_1*:*Default';
  | 
  | %Inertia Type - Custom
  | %Visual Properties - Simple
  | smiData.Solid(3).mass = 0.0018077786468980381;  % kg
  | smiData.Solid(3).CoM = [19.27726280951001 -0.0039942113333676097 6.8843889734069202e-07];  % mm
  | smiData.Solid(3).MoI = [0.019566370524392956 0.25748886727483228 0.25011722572433198];  % kg*mm^2
  | smiData.Solid(3).PoI = [-3.0141334312561118e-09 -1.3904563423966734e-08 0.00012612854914179953];  % kg*mm^2
  | smiData.Solid(3).color = [0.792156862745098 0.81960784313725488 0.93333333333333335];
  | smiData.Solid(3).opacity = 1;
  | smiData.Solid(3).ID = 'Joint_2*:*Default';
  | 
  | %Inertia Type - Custom
  | %Visual Properties - Simple
  | smiData.Solid(4).mass = 0.017070467811714975;  % kg
  | smiData.Solid(4).CoM = [-1.5772967019100965e-11 -5.5159552640168081e-13 0];  % mm
  | smiData.Solid(4).MoI = [0.2846003979118012 186.94882272197759 186.94882272197759];  % kg*mm^2
  | smiData.Solid(4).PoI = [0 0 0];  % kg*mm^2
  | smiData.Solid(4).color = [0.792156862745098 0.81960784313725488 0.93333333333333335];
  | smiData.Solid(4).opacity = 1;
  | smiData.Solid(4).ID = 'Lower_Leg*:*Default';
  | 
  | %Inertia Type - Custom
  | %Visual Properties - Simple
  | smiData.Solid(5).mass = 0.021488486382231504;  % kg
  | smiData.Solid(5).CoM = [14.546414891457909 12.467715063250926 25];  % mm
  | smiData.Solid(5).MoI = [8.6594151200892373 9.6419513792455867 9.1654649617944717];  % kg*mm^2
  | smiData.Solid(5).PoI = [0 0 2.5503965876805252];  % kg*mm^2
  | smiData.Solid(5).color = [0.792156862745098 0.81960784313725488 0.93333333333333335];
  | smiData.Solid(5).opacity = 1;
  | smiData.Solid(5).ID = 'Gá_cho_Upper_Leg*:*Default';
  | 
  | %Inertia Type - Custom
  | %Visual Properties - Simple
  | smiData.Solid(6).mass = 6.0518207712728707;  % kg
  | smiData.Solid(6).CoM = [349.99999999999972 14.999999999999996 -202.07259421636917];  % mm
  | smiData.Solid(6).MoI = [126619.22609403533 252330.67907237998 126619.22609403556];  % kg*mm^2
  | smiData.Solid(6).PoI = [0 0 0];  % kg*mm^2
  | smiData.Solid(6).color = [0.792156862745098 0.81960784313725488 0.93333333333333335];
  | smiData.Solid(6).opacity = 1;
  | smiData.Solid(6).ID = 'M?t_Base*:*Default';
  | 
  | %Inertia Type - Custom
  | %Visual Properties - Simple
  | smiData.Solid(7).mass = 0.00078539816339744757;  % kg
  | smiData.Solid(7).CoM = [5.0000000000000018 0 0];  % mm
  | smiData.Solid(7).MoI = [0.0098174770424680861 0.011453723216212772 0.011453723216212772];  % kg*mm^2
  | smiData.Solid(7).PoI = [0 0 0];  % kg*mm^2
  | smiData.Solid(7).color = [0.792156862745098 0.81960784313725488 0.93333333333333335];
  | smiData.Solid(7).opacity = 1;
  | smiData.Solid(7).ID = 'x?*:*Default';
  | 
  | %Inertia Type - Custom
  | %Visual Properties - Simple
  | smiData.Solid(8).mass = 0.10295887995248661;  % kg
  | smiData.Solid(8).CoM = [0 9.8031105328807815 0];  % mm
  | smiData.Solid(8).MoI = [94.641180461165206 181.81625552883975 94.641180461165234];  % kg*mm^2
  | smiData.Solid(8).PoI = [0 0 0];  % kg*mm^2
  | smiData.Solid(8).color = [0.792156862745098 0.81960784313725488 0.93333333333333335];
  | smiData.Solid(8).opacity = 1;
  | smiData.Solid(8).ID = '�?*:*Default';
  | 
  | 
  | %============= Joint =============%
  | %X Revolute Primitive (Rx) %Y Revolute Primitive (Ry) %Z Revolute Primitive (Rz)
  | %X Prismatic Primitive (Px) %Y Prismatic Primitive (Py) %Z Prismatic Primitive (Pz) %Spherical Primitive (S)
  | %Constant Velocity Primitive (CV) %Lead Screw Primitive (LS)
  | %Position Target (Pos)
  | 
  | %Initialize the CylindricalJoint structure array by filling in null values.
  | smiData.CylindricalJoint(3).Rz.Pos = 0.0;
  | smiData.CylindricalJoint(3).Pz.Pos = 0.0;
  | smiData.CylindricalJoint(3).ID = '';
  | 
  | smiData.CylindricalJoint(1).Rz.Pos = -96.649707795084993;  % deg
  | smiData.CylindricalJoint(1).Pz.Pos = 0;  % mm
  | smiData.CylindricalJoint(1).ID = '[LowerLeg_Assembly#2-2:-:x?-10]';
  | 
  | smiData.CylindricalJoint(2).Rz.Pos = -65.651337876243986;  % deg
  | smiData.CylindricalJoint(2).Pz.Pos = 0;  % mm
  | smiData.CylindricalJoint(2).ID = '[LowerLeg_Assembly#2-4:-:x?-2]';
  | 
  | smiData.CylindricalJoint(3).Rz.Pos = -65.651337877337426;  % deg
  | smiData.CylindricalJoint(3).Pz.Pos = 0;  % mm
  | smiData.CylindricalJoint(3).ID = '[LowerLeg_Assembly#2-4:-:x?-3]';
  | 
  | 
  | %Initialize the PlanarJoint structure array by filling in null values.
  | smiData.PlanarJoint(3).Rz.Pos = 0.0;
  | smiData.PlanarJoint(3).Px.Pos = 0.0;
  | smiData.PlanarJoint(3).Py.Pos = 0.0;
  | smiData.PlanarJoint(3).ID = '';
  | 
  | %This joint has been chosen as a cut joint. Simscape Multibody treats cut joints as algebraic constraints to solve closed kinematic loops. The imported model does not use the state target data for this joint.
  | smiData.PlanarJoint(1).Rz.Pos = -170.63129784075477;  % deg
  | smiData.PlanarJoint(1).Px.Pos = 0;  % mm
  | smiData.PlanarJoint(1).Py.Pos = 0;  % mm
  | smiData.PlanarJoint(1).ID = '[UpperLeg_2-3:Joint_1-1:-:x?-10]';
  | 
  | %This joint has been chosen as a cut joint. Simscape Multibody treats cut joints as algebraic constraints to solve closed kinematic loops. The imported model does not use the state target data for this joint.
  | smiData.PlanarJoint(2).Rz.Pos = 36.138428467299015;  % deg
  | smiData.PlanarJoint(2).Px.Pos = 0;  % mm
  | smiData.PlanarJoint(2).Py.Pos = 0;  % mm
  | smiData.PlanarJoint(2).ID = '[UpperLeg_2-4:Joint_1-1:-:x?-2]';
  | 
  | %This joint has been chosen as a cut joint. Simscape Multibody treats cut joints as algebraic constraints to solve closed kinematic loops. The imported model does not use the state target data for this joint.
  | smiData.PlanarJoint(3).Rz.Pos = -143.86157153379796;  % deg
  | smiData.PlanarJoint(3).Px.Pos = 0;  % mm
  | smiData.PlanarJoint(3).Py.Pos = 0;  % mm
  | smiData.PlanarJoint(3).ID = '[Base_3-1:Joint_1-4:-:x?-3]';
  | 
  | 
  | %Initialize the RevoluteJoint structure array by filling in null values.
  | smiData.RevoluteJoint(30).Rz.Pos = 0.0;
  | smiData.RevoluteJoint(30).ID = '';
  | 
  | smiData.RevoluteJoint(1).Rz.Pos = 178.28499306347177;  % deg
  | smiData.RevoluteJoint(1).ID = '[UpperLeg_2-3:Upper_Leg-1:-:UpperLeg_2-3:Joint_1-1]';
  | 
  | smiData.RevoluteJoint(2).Rz.Pos = -10.034581161452214;  % deg
  | smiData.RevoluteJoint(2).ID = '[UpperLeg_2-4:Upper_Leg-1:-:UpperLeg_2-4:Joint_1-1]';
  | 
  | smiData.RevoluteJoint(3).Rz.Pos = -167.53904085225858;  % deg
  | smiData.RevoluteJoint(3).ID = '[UpperLeg_2-5:Upper_Leg-1:-:UpperLeg_2-5:Joint_1-1]';
  | 
  | smiData.RevoluteJoint(4).Rz.Pos = -137.92683463517784;  % deg
  | smiData.RevoluteJoint(4).ID = '[Base_3-1:�?-1:-:Base_3-1:Joint_1-1]';
  | 
  | %This joint has been chosen as a cut joint. Simscape Multibody treats cut joints as algebraic constraints to solve closed kinematic loops. The imported model does not use the state target data for this joint.
  | smiData.RevoluteJoint(5).Rz.Pos = -141.04967383445427;  % deg
  | smiData.RevoluteJoint(5).ID = '[Base_3-1:�?-1:-:Base_3-1:Joint_1-4]';
  | 
  | %This joint has been chosen as a cut joint. Simscape Multibody treats cut joints as algebraic constraints to solve closed kinematic loops. The imported model does not use the state target data for this joint.
  | smiData.RevoluteJoint(6).Rz.Pos = -63.307207190855458;  % deg
  | smiData.RevoluteJoint(6).ID = '[Base_3-1:�?-1:-:Base_3-1:Joint_1-5]';
  | 
  | smiData.RevoluteJoint(7).Rz.Pos = -6.7114691797928572;  % deg
  | smiData.RevoluteJoint(7).ID = '[UpperLeg_2-5:Joint_1-1:-:x?-11]';
  | 
  | smiData.RevoluteJoint(8).Rz.Pos = -6.711469179624248;  % deg
  | smiData.RevoluteJoint(8).ID = '[UpperLeg_2-5:Joint_1-1:-:x?-12]';
  | 
  | smiData.RevoluteJoint(9).Rz.Pos = -54.534124512986644;  % deg
  | smiData.RevoluteJoint(9).ID = '[Base-1:-:UpperLeg_2-5:Upper_Leg-1]';
  | 
  | smiData.RevoluteJoint(10).Rz.Pos = 87.281005635845503;  % deg
  | smiData.RevoluteJoint(10).ID = '[LowerLeg_Assembly#2-1:-:Base_3-1:Joint_1-5]';
  | 
  | smiData.RevoluteJoint(11).Rz.Pos = -92.718994364160224;  % deg
  | smiData.RevoluteJoint(11).ID = '[UpperLeg_2-3:Joint_1-1:-:LowerLeg_Assembly#2-1]';
  | 
  | %This joint has been chosen as a cut joint. Simscape Multibody treats cut joints as algebraic constraints to solve closed kinematic loops. The imported model does not use the state target data for this joint.
  | smiData.RevoluteJoint(12).Rz.Pos = 87.281005635845489;  % deg
  | smiData.RevoluteJoint(12).ID = '[LowerLeg_Assembly#2-2:-:Base_3-1:Joint_1-5]';
  | 
  | smiData.RevoluteJoint(13).Rz.Pos = -92.718994364160267;  % deg
  | smiData.RevoluteJoint(13).ID = '[UpperLeg_2-3:Joint_1-1:-:LowerLeg_Assembly#2-2]';
  | 
  | smiData.RevoluteJoint(14).Rz.Pos = 78.210233656460574;  % deg
  | smiData.RevoluteJoint(14).ID = '[LowerLeg_Assembly#2-3:-:Base_3-1:Joint_1-4]';
  | 
  | smiData.RevoluteJoint(15).Rz.Pos = -101.78976634354296;  % deg
  | smiData.RevoluteJoint(15).ID = '[UpperLeg_2-4:Joint_1-1:-:LowerLeg_Assembly#2-3]';
  | 
  | %This joint has been chosen as a cut joint. Simscape Multibody treats cut joints as algebraic constraints to solve closed kinematic loops. The imported model does not use the state target data for this joint.
  | smiData.RevoluteJoint(16).Rz.Pos = 78.210233656460517;  % deg
  | smiData.RevoluteJoint(16).ID = '[LowerLeg_Assembly#2-4:-:Base_3-1:Joint_1-4]';
  | 
  | smiData.RevoluteJoint(17).Rz.Pos = -101.78976634354302;  % deg
  | smiData.RevoluteJoint(17).ID = '[UpperLeg_2-4:Joint_1-1:-:LowerLeg_Assembly#2-4]';
  | 
  | smiData.RevoluteJoint(18).Rz.Pos = -80.973943718088847;  % deg
  | smiData.RevoluteJoint(18).ID = '[LowerLeg_Assembly#2-5:-:Base_3-1:Joint_1-1]';
  | 
  | %This joint has been chosen as a cut joint. Simscape Multibody treats cut joints as algebraic constraints to solve closed kinematic loops. The imported model does not use the state target data for this joint.
  | smiData.RevoluteJoint(19).Rz.Pos = -80.97394371808717;  % deg
  | smiData.RevoluteJoint(19).ID = '[LowerLeg_Assembly#2-6:-:Base_3-1:Joint_1-1]';
  | 
  | smiData.RevoluteJoint(20).Rz.Pos = -41.015092672769711;  % deg
  | smiData.RevoluteJoint(20).ID = '[Base-1:-:UpperLeg_2-4:Upper_Leg-1]';
  | 
  | smiData.RevoluteJoint(21).Rz.Pos = -151.59220025492431;  % deg
  | smiData.RevoluteJoint(21).ID = '[Base-1:-:UpperLeg_2-3:Upper_Leg-1]';
  | 
  | smiData.RevoluteJoint(22).Rz.Pos = 80.973943718091775;  % deg
  | smiData.RevoluteJoint(22).ID = '[UpperLeg_2-5:Joint_1-1:-:LowerLeg_Assembly#2-5]';
  | 
  | smiData.RevoluteJoint(23).Rz.Pos = 80.973943718090084;  % deg
  | smiData.RevoluteJoint(23).ID = '[UpperLeg_2-5:Joint_1-1:-:LowerLeg_Assembly#2-6]';
  | 
  | smiData.RevoluteJoint(24).Rz.Pos = 23.780653335597517;  % deg
  | smiData.RevoluteJoint(24).ID = '[UpperLeg_2-4:Joint_1-1:-:x?-1]';
  | 
  | smiData.RevoluteJoint(25).Rz.Pos = -156.21934666376924;  % deg
  | smiData.RevoluteJoint(25).ID = '[Base_3-1:Joint_1-4:-:x?-4]';
  | 
  | smiData.RevoluteJoint(26).Rz.Pos = -7.0798145757958322;  % deg
  | smiData.RevoluteJoint(26).ID = '[Base_3-1:Joint_1-1:-:x?-5]';
  | 
  | smiData.RevoluteJoint(27).Rz.Pos = -7.0798145757073732;  % deg
  | smiData.RevoluteJoint(27).ID = '[Base_3-1:Joint_1-1:-:x?-6]';
  | 
  | smiData.RevoluteJoint(28).Rz.Pos = -172.77668326833376;  % deg
  | smiData.RevoluteJoint(28).ID = '[Base_3-1:Joint_1-5:-:x?-7]';
  | 
  | smiData.RevoluteJoint(29).Rz.Pos = -172.77668326853527;  % deg
  | smiData.RevoluteJoint(29).ID = '[Base_3-1:Joint_1-5:-:x?-8]';
  | 
  | smiData.RevoluteJoint(30).Rz.Pos = -7.043414688128661;  % deg
  | smiData.RevoluteJoint(30).ID = '[UpperLeg_2-3:Joint_1-1:-:x?-9]';
undefined symbols (not defined in the file): DiscIntNeverNeededParam, smiData, X, Y, Z
libraries: sm_lib x246, nesl_utility x13
(part 1 of 6)
settings Model: Creator=FPTSHOP  LastModifiedBy=FPTSHOP

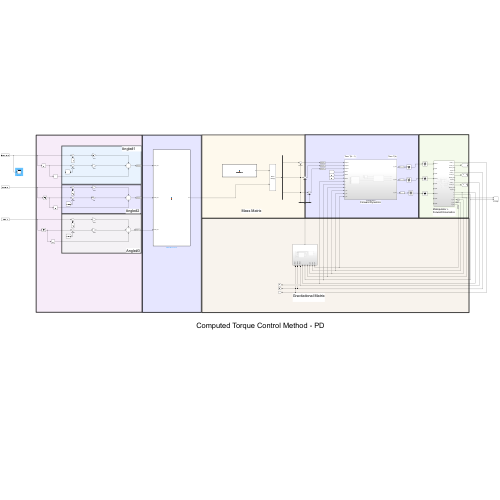
[thumbnail: Simulink's stored preview of the top-level diagram]
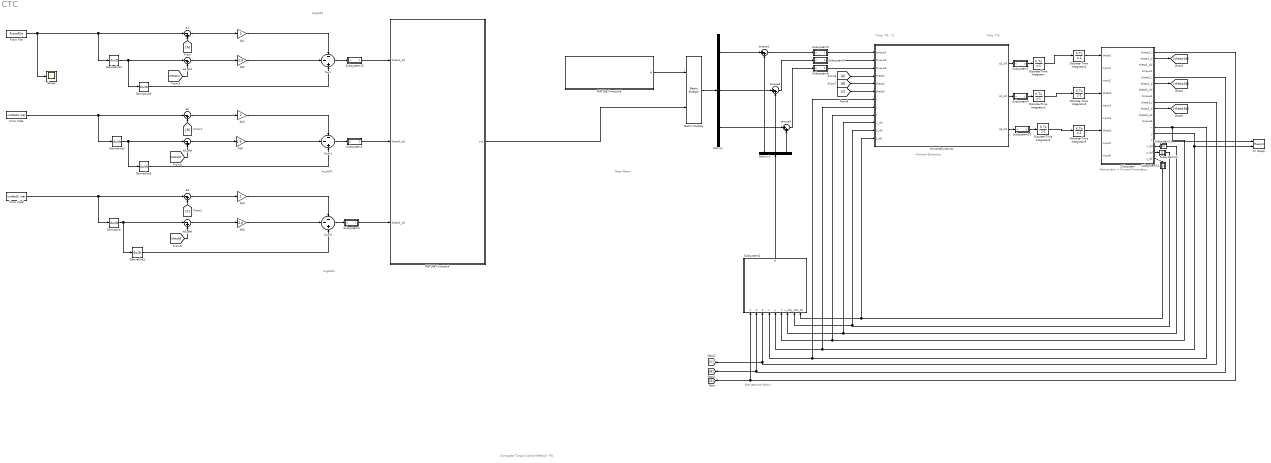
== system CTC ==
  note: Computed Torque Control Method - PD
  note: Malnipulator + Forward Kinematics
  note: Forward Dynamics
  note: Time: T(k - 1)
  note: Time: T(k)
  note: Gravitational Matrix
  note: Mass Matrix
  note: Angle#1
  note: Angle#2
  note: Angle#3
  Demux : Demux  Outputs=3
  Demux1 : Demux  Outputs=3
  Derivative{,1..5} (6 alike) : Derivative
  Discrete-Time Integrator{,1..5} (6 alike) : DiscreteIntegrator  SampleTime=0.01  ICPrevOutput=DiscIntNeverNeededParam  ICPrevScaledInput=DiscIntNeverNeededParam
  From : From
  From File : FromFile  SampleTime=0
  From File1 : FromFile  FileName=untitled1.mat  SampleTime=0
  From File2 : FromFile  FileName=untitled2.mat  SampleTime=0
  From6 : From
  Goto : Goto
  Kd1 : Gain  Gain=2.6
  Kd2 : Gain  Gain=2.6
  Kd3 : Gain  Gain=2.6
  Kp1 : Gain  Gain=2
  Kp2 : Gain  Gain=2
  Kp3 : Gain  Gain=2
  MATLAB Function3 : MATLAB Function  TreatAsAtomicUnit=on
  MATLAB Function5 : MATLAB Function  TreatAsAtomicUnit=on
  Matrix Multiply : Product  Multiplication=Matrix(*)
  Scope : Scope
  Subsystem : Subsystem
  Subsystem1 : Subsystem
  Subsystem10 : Subsystem
  Subsystem11 : Subsystem
  Subsystem12 : Subsystem
  Subsystem13 : Subsystem
  Subsystem14 : Subsystem
  Subsystem2 : Subsystem
  Subsystem3 : Subsystem
  Subsystem5 : Subsystem
  Subsystem6 : Subsystem
  Subsystem7 : Subsystem
  Subsystem8 : Subsystem
  Subsystem9 : Subsystem
  Sum : Sum  Inputs=--+
  Sum1 : Sum  Inputs=--+
  Sum2 : Sum  Inputs=--+
  XY Graph : Record  FileSettingsInternal="{\"entries\":[{\"content\":{\"excelSettings\":{\"content\":{},\"type\":\"Streamout.ExcelSettings\"}},\"type\":\"Streamout.FileSettingStorage\",\"uuid\":\"be05fd02-d853-4528-90b8-9b4994329b9c\"}],\"packageUris\":[\"http://schema.mathworks.com/mf0/streamout_blocks/R2020a\"],\"version\":\"1.0\"}"  Layout=[1 1]  SignalsInternal="{\"entries\":[{\"content\":{\"signals\":[{\"content\":{\"blockPath\":[\"CTC/XY Graph\"],\"channel\":[],\"dimensions\":[1],\"domain\":\"CTC/XY Graph\",\"lineColor\":\"#a2142f\",\"plots\":[1],\"port\":1,\"sid\":[\"\"],\"signalID\":341,\"signalName\":\"Subsystem:13\"},\"type\":\"RecordBlkView.Signal\",\"uuid\":\"32d67d64-25e4-4189-abcd-9f6079fd6c20\"},{\"content\":{\"blockPath\":[\"CTC/XY Graph\"],\"channel\":[],\"dimensions\":[1],\"domain\":\"CTC/XY Graph\",\"lineColor\":\"#139fff\",\"plots\":[1],\"port\":2,\"sid\":[\"\"],\"signalID\":345,\"signalName\":\"Subsystem:14\"},\"type\":\"RecordBlkView.Signal\",\"uuid\":\"b8ee85d2-38ce-4b4c-99af-7bae53f07012\"}]},\"type\":\"RecordBlkView.InputSignals\",\"uuid\":\"056bfb51-bee3-4825-a7ce-a2bcfe8fb366\"}],\"packageUris\":[\"http://schema.mathworks.com/mf0/streamout_blocks/R2020a\"],\"version\":\"1.0\"}"  VisualizationBindings="{\"xyplotplugin\":{\"info\":[{\"series\":[{\"bindingParametersList\":[{\"parameter\":\"X-Axis\",\"signalID\":341,\"signalName\":\"Subsystem:13\"},{\"parameter\":\"Y-Axis\",\"signalID\":345,\"signalName\":\"Subsystem:14\"}],\"seriesID\":57718}],\"subplotID\":1}]}}"  CompatibilityTag=XY
  e1 : Sum  Inputs=|-+
  e1_dot : Sum  Inputs=|-+
  e2 : Sum  Inputs=|-+
  e2_dot : Sum  Inputs=|-+
  e3 : Sum  Inputs=|-+
  e3_dot : Sum  Inputs=|-+
  forwardDynamics : Subsystem
  torque1 : Sum  Inputs=|++
  torque2 : Sum  Inputs=|++
  torque3 : Sum  Inputs=|++
  wires:
  Discrete-Time Integrator1/1 -> Subsystem/1(theta1)
  forwardDynamics/1(q1_dd) -> Subsystem7/1(u)
  Discrete-Time Integrator/1 -> Discrete-Time Integrator1/1
  forwardDynamics/2(q2_dd) -> Subsystem9/1(u)
  Discrete-Time Integrator3/1 -> Subsystem/4(theta2)
  Discrete-Time Integrator2/1 -> Discrete-Time Integrator3/1
  Discrete-Time Integrator5/1 -> Subsystem/7(theta3)
  Discrete-Time Integrator4/1 -> Discrete-Time Integrator5/1
  forwardDynamics/3(q3_dd) -> Subsystem10/1(u)
  Demux1/3 -> torque3/2
  Demux/2 -> torque2/1
  Subsystem2/1(G) -> Demux1/1
  Demux/1 -> torque1/1
  Demux1/1 -> torque1/2
  Matrix Multiply/1 -> Demux/1
  Demux/3 -> torque3/1
  Demux1/2 -> torque2/2
  MATLAB Function5/1(M) -> Matrix Multiply/1
  torque1/1 -> Subsystem5/1(u)
  torque2/1 -> Subsystem6/1(u)
  torque3/1 -> Subsystem8/1(u)
  Subsystem/15(z) -> forwardDynamics/9(z), Subsystem2/6(z)
  Subsystem/14(y) -> XY Graph/2, forwardDynamics/8(y), Subsystem2/5(y)
  Subsystem/13(x) -> XY Graph/1, forwardDynamics/7(x), Subsystem2/4(x)
  Subsystem/9(theta3_r) -> [C], Subsystem2/3(theta3)
  Subsystem/5(theta2_r) -> [B], Subsystem2/2(theta2)
  Subsystem/1(theta1_r) -> Subsystem2/1(theta1), Goto/1
  Kp1/1 -> Sum/1
  e2/1 -> Kp2/1
  e3_dot/1 -> Kd3/1
  e2_dot/1 -> Kd2/1
  Kd3/1 -> Sum2/2
  Kp2/1 -> Sum1/1
  Kp3/1 -> Sum2/1
  Kd2/1 -> Sum1/2
  e1_dot/1 -> Kd1/1
  Kd1/1 -> Sum/2
  e1/1 -> Kp1/1
  e3/1 -> Kp3/1
  Sum2/1 -> Subsystem3/1(u)
  Sum1/1 -> Subsystem1/1(u)
  Sum/1 -> Subsystem13/1(u)
  MATLAB Function3/1(out) -> Matrix Multiply/2
  From/1 -> e1/2
  [B] -> e2/2
  [C] -> e3/2
  Subsystem/2(theta1_d) -> [theta1d]
  Subsystem/6(theta2_d) -> [theta2d]
  Subsystem/10(theta3_d) -> [theta3d]
  [theta1d] -> e1_dot/2
  [theta2d] -> e2_dot/2
  [theta3d] -> e3_dot/2
  Derivative/1 -> Derivative1/1, e3_dot/1
  Derivative1/1 -> Sum2/3
  Derivative2/1 -> Derivative3/1, e2_dot/1
  Derivative3/1 -> Sum1/3
  Derivative4/1 -> e1_dot/1, Derivative5/1
  Derivative5/1 -> Sum/3
  Subsystem13/1(torque1) -> MATLAB Function3/1(theta1_dd)
  Subsystem1/1(torque1) -> MATLAB Function3/2(theta2_dd)
  Subsystem3/1(torque1) -> MATLAB Function3/3(theta3_dd)
  Subsystem/18(z_dd) -> Subsystem14/1(u)
  Subsystem/17(y_dd) -> Subsystem12/1(u)
  Subsystem/16(x_dd) -> Subsystem11/1(u)
  From6/1 -> forwardDynamics/4(theta1)
  [B] -> forwardDynamics/5(theta2)
  [C] -> forwardDynamics/6(theta3)
  Subsystem7/1(y) -> Discrete-Time Integrator/1
  Subsystem9/1(y) -> Discrete-Time Integrator2/1
  Subsystem10/1(y) -> Discrete-Time Integrator4/1
  Subsystem11/1(y) -> forwardDynamics/10(x_dd), Subsystem2/7(x_dd)
  Subsystem12/1(y) -> forwardDynamics/11(y_dd), Subsystem2/8(y_dd)
  Subsystem14/1(y) -> forwardDynamics/12(z_dd), Subsystem2/9(z_dd)
  From File/1 -> Scope/1, Derivative4/1, e1/1
  From File1/1 -> Derivative2/1, e2/1
  From File2/1 -> Derivative/1, e3/1
  Subsystem6/1(torque1) -> forwardDynamics/2(torque2)
  Subsystem8/1(torque1) -> forwardDynamics/3(torque3)
  Subsystem5/1(torque1) -> forwardDynamics/1(torque1)
